simulink model "validacion_LTI"  (R2023b)
settings: Solver=VariableStepAuto  StartTime=0.0  StopTime=10.0  RelTol=1e-3
PostLoadFcn:
  | parametros_sistema_completo
  | run("parametros_sistema_completo.mlx")
values from neighbouring files (symbols this model uses):
  a_cu = 3.9e-3    (= 0.0039)    [parametros_sistema_completo.m]    (also in workspace_params.mat)
  A_sim = sys_design.A    [generar_modelo_LTI.m]
  b_eq = params.b_total    [calcular_matriz_AO.m]    (also in calculo_incertidumbre_y_control.m = b_m + b_l/(r^2); parametros_sistema_completo.m = 2.19444444444e-05; workspace_params.mat = 2.19444444444e-05)
  B_sim = sys_design.B    [generar_modelo_LTI.m]
  C_sim = eye(6)    [generar_modelo_LTI.m]
  C_ts = C_ts * (1 + tol_pct)    [calculo_incertidumbre_y_control.m]    (also in parametros_sistema_completo.m = 0.818; workspace_params.mat = 0.818)
  D_sim = zeros(6,3)    [generar_modelo_LTI.m]
  g = 9.80665    [parametros_sistema_completo.m]    (also in workspace_params.mat)
  J_eq = params.J_total    [calcular_matriz_AO.m]    (also in calculo_incertidumbre_y_control.m = J_m + J_l/r^2; parametros_sistema_completo.m = 1.97847222222e-05; workspace_params.mat = 3.28055555556e-05)
  k_l = m*l_cm + m_l*l_l    [calculo_incertidumbre_y_control.m]    (also in parametros_sistema_completo.m = 0.25; workspace_params.mat = 0.625)
  L_d = L_d    * (1 - tol_pct)    [calculo_incertidumbre_y_control.m]    (also in parametros_sistema_completo.m = 0.0066; workspace_params.mat = 0.0066)
  L_ls = L_ls   * (1 - tol_pct)    [calculo_incertidumbre_y_control.m]    (also in parametros_sistema_completo.m = 0.0008; workspace_params.mat = 0.0008)
  L_q = L_q    * (1 - tol_pct)    [calculo_incertidumbre_y_control.m]    (also in parametros_sistema_completo.m = 0.0058; workspace_params.mat = 0.0058)
  lambda_r = lambda_r * (1 + tol_pct)    [calculo_incertidumbre_y_control.m]    (also in parametros_sistema_completo.m = 0.016; workspace_params.mat = 0.016)
  P_p = 3    [parametros_sistema_completo.m]    (also in workspace_params.mat)
  r = params.r_red    [calcular_matriz_AO.m]    (also in parametros_sistema_completo.m = 120; workspace_params.mat = 120)
  R_sREF = R_sREF * (1 - tol_pct)    [calculo_incertidumbre_y_control.m]    (also in parametros_sistema_completo.m = 1.02; workspace_params.mat = 1.02)
  R_ts_amb = R_ts_amb * (1 - tol_pct)    [calculo_incertidumbre_y_control.m]    (also in parametros_sistema_completo.m = 146.7; workspace_params.mat = 146.7)
  T_amb = 20    [parametros_sistema_completo.m]    (also in workspace_params.mat)
  T_sREF = 20    [parametros_sistema_completo.m]    (also in workspace_params.mat)
  val_th_m_90 = val_th_l_90 * r    [generar_modelo_LTI.m]
settings Model: Creator=Francisco  LastModifiedBy=calde
settings DebuggingCC: UnderspecifiedInitializationDetection=Classic  MergeDetectMultiDrivingBlocksExec=none
settings ModelReferenceCC: PropagateSignalLabelsOutOfModel=off

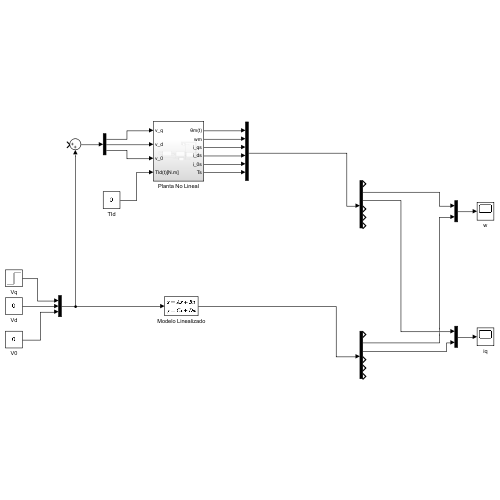
[thumbnail: Simulink's stored preview of the top-level diagram]
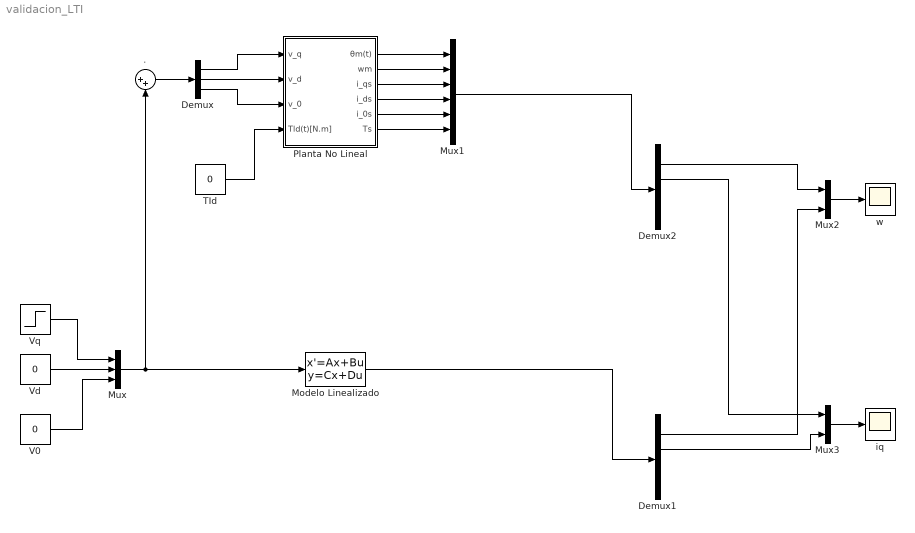
== system validacion_LTI ==
  . : Sum  Inputs=|++
  Demux : Demux  Outputs=3
  Demux1 : Demux  Outputs=6
  Demux2 : Demux  Outputs=6
  Modelo Linealizado : StateSpace  A=A_sim  B=B_sim  C=C_sim  D=D_sim  InitialCondition=0
  Mux : Mux  Inputs=3
  Mux1 : Mux  Inputs=6
  Mux2 : Mux  Inputs=2
  Mux3 : Mux  Inputs=2
  Planta No Lineal : Subsystem
  TId : Constant  Value=0
  V0 : Constant  Value=0
  Vd : Constant  Value=0
  Vq : Step  Time=0.5  SampleTime=0
  iq : Scope
  w : Scope
  wires:
  TId/1 -> Planta No Lineal/4(Tld(t)[N.m])
  Vq/1 -> Mux/1
  Vd/1 -> Mux/2
  V0/1 -> Mux/3
  Mux/1 -> Modelo Linealizado/1, ./2
  ./1 -> Demux/1
  Demux/1 -> Planta No Lineal/1(v_q)
  Demux/2 -> Planta No Lineal/2(v_d)
  Demux/3 -> Planta No Lineal/3(v_0)
  Planta No Lineal/1(θm(t)) -> Mux1/1
  Planta No Lineal/2(wm) -> Mux1/2
  Planta No Lineal/3(i_qs) -> Mux1/3
  Planta No Lineal/4(i_ds) -> Mux1/4
  Planta No Lineal/5(i_0s) -> Mux1/5
  Planta No Lineal/6(Ts) -> Mux1/6
  Mux1/1 -> Demux2/1
  Demux2/2 -> Mux2/1
  Demux2/3 -> Mux3/1
  Demux1/2 -> Mux2/2
  Demux1/3 -> Mux3/2
  Mux2/1 -> w/1
  Mux3/1 -> iq/1
  Modelo Linealizado/1 -> Demux1/1

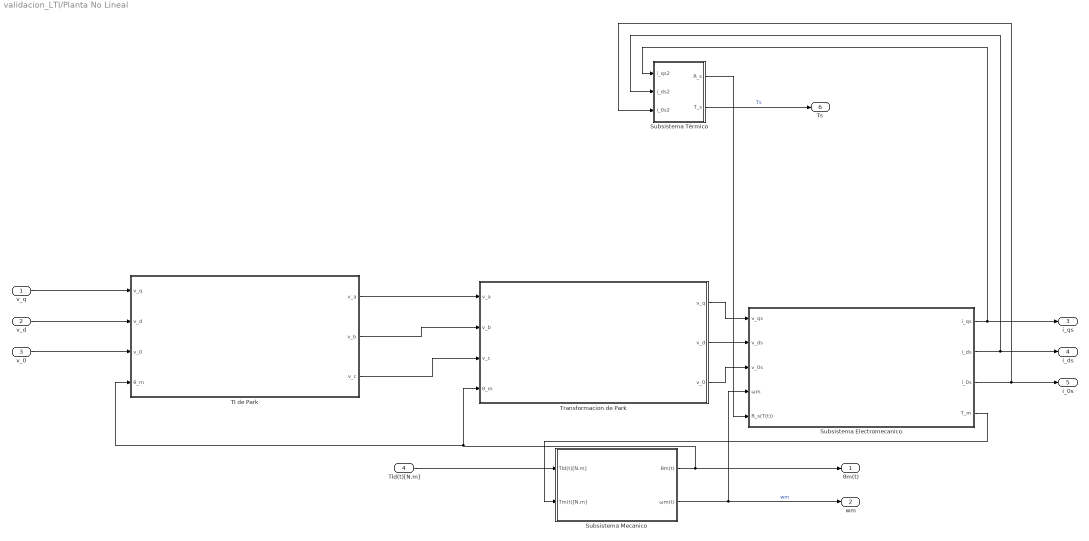
== system validacion_LTI/Planta No Lineal ==
  v_q : Inport
  v_d : Inport  Port=2
  v_0 : Inport  Port=3
  Tld(t)[N.m] : Inport  Port=4
  Subsistema Electromecanico : Subsystem
  Subsistema Mecanico : Subsystem
  Subsistema Térmico : Subsystem
  TI de Park : Subsystem
  Transformacion de Park : Subsystem
  θm(t) : Outport
  wm : Outport  Port=2
  i_qs : Outport  Port=3
  i_ds : Outport  Port=4
  i_0s : Outport  Port=5
  Ts : Outport  Port=6
  wires:
  TI de Park/1(v_a) -> Transformacion de Park/1(v_a)
  TI de Park/3(v_c) -> Transformacion de Park/3(v_c)
  Transformacion de Park/1(v_q) -> Subsistema Electromecanico/1(v_qs)
  TI de Park/2(v_b) -> Transformacion de Park/2(v_b)
  Subsistema Electromecanico/4(T_m) -> Subsistema Mecanico/2(Tm(t)[N.m])
  Subsistema Electromecanico/2(i_ds) -> i_ds/1, Subsistema Térmico/2(i_ds2)
  Subsistema Mecanico/1(θm(t)) -> θm(t)/1, TI de Park/4(θ_m), Transformacion de Park/4(θ_m)
  Subsistema Electromecanico/3(i_0s) -> i_0s/1, Subsistema Térmico/3(i_0s2)
  Subsistema Mecanico/2(ωm(t)) -> wm/1, Subsistema Electromecanico/4(ωm)  "wm"
  Subsistema Térmico/1(R_s) -> Subsistema Electromecanico/5(R_s(T(t)))
  Transformacion de Park/3(v_0) -> Subsistema Electromecanico/3(v_0s)
  Transformacion de Park/2(v_d) -> Subsistema Electromecanico/2(v_ds)
  Subsistema Electromecanico/1(i_qs) -> i_qs/1, Subsistema Térmico/1(i_qs2)
  v_q/1 -> TI de Park/1(v_q)
  v_d/1 -> TI de Park/2(v_d)
  Tld(t)[N.m]/1 -> Subsistema Mecanico/1(Tld(t)[N.m])
  v_0/1 -> TI de Park/3(v_0)
  Subsistema Térmico/2(T_s) -> Ts/1  "Ts"

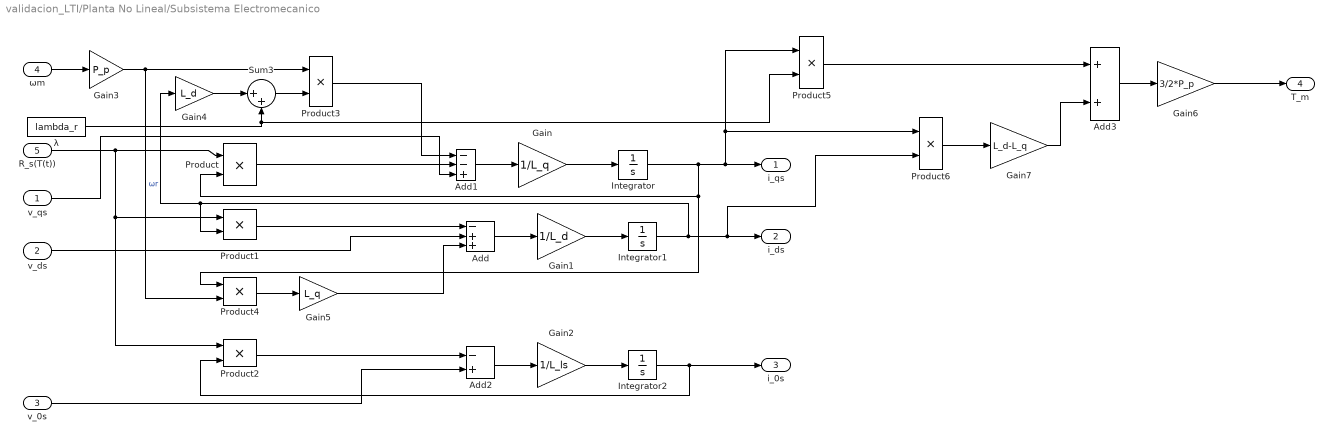
== system validacion_LTI/Planta No Lineal/Subsistema Electromecanico ==
  v_qs : Inport
  v_ds : Inport  Port=2
  v_0s : Inport  Port=3
  ωm : Inport  Port=4
  R_s(T(t)) : Inport  Port=5
  Add : Sum  Inputs=-++
  Add1 : Sum  Inputs=--+
  Add2 : Sum  Inputs=-+
  Add3 : Sum
  Gain : Gain  Gain=1/L_q
  Gain1 : Gain  Gain=1/L_d
  Gain2 : Gain  Gain=1/L_ls
  Gain3 : Gain  Gain=P_p
  Gain4 : Gain  Gain=L_d
  Gain5 : Gain  Gain=L_q
  Gain6 : Gain  Gain=3/2*P_p
  Gain7 : Gain  Gain=L_d-L_q
  Integrator : Integrator
  Integrator1 : Integrator
  Integrator2 : Integrator
  Product{,1..6} (7 alike) : Product
  Sum3 : Sum  Inputs=|++
  λ : Constant  Value=lambda_r
  i_qs : Outport
  i_ds : Outport  Port=2
  i_0s : Outport  Port=3
  T_m : Outport  Port=4
  wires:
  v_0s/1 -> Add2/2
  Gain5/1 -> Add/3
  Gain3/1 -> Product4/2, Product3/1  "ωr"
  Integrator/1 -> Product4/1, Product/2, i_qs/1, Product5/1, Product6/1
  v_qs/1 -> Add1/3
  R_s(T(t))/1 -> Product2/1, Product1/1, Product/1
  Gain4/1 -> Sum3/1
  Product1/1 -> Add/1
  Integrator2/1 -> i_0s/1, Product2/2
  Sum3/1 -> Product3/2
  Integrator1/1 -> Gain4/1, Product1/2, i_ds/1, Product6/2
  Product/1 -> Add1/2
  Product4/1 -> Gain5/1
  ωm/1 -> Gain3/1
  Add3/1 -> Gain6/1
  Gain/1 -> Integrator/1
  Gain6/1 -> T_m/1
  Product2/1 -> Add2/1
  λ/1 -> Sum3/2, Product5/2
  Gain1/1 -> Integrator1/1
  Add/1 -> Gain1/1
  Add1/1 -> Gain/1
  Product6/1 -> Gain7/1
  Product3/1 -> Add1/1
  Gain2/1 -> Integrator2/1
  Gain7/1 -> Add3/2
  v_ds/1 -> Add/2
  Add2/1 -> Gain2/1
  Product5/1 -> Add3/1

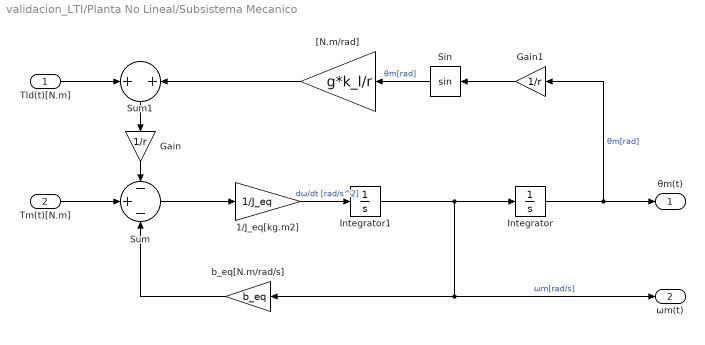
== system validacion_LTI/Planta No Lineal/Subsistema Mecanico ==
  Tld(t)[N.m] : Inport
  Tm(t)[N.m] : Inport  Port=2
  1/J_eq[kg.m2] : Gain  Gain=1/J_eq
  Gain : Gain  Gain=1/r
  Gain1 : Gain  Gain=1/r
  Integrator : Integrator  InitialCondition=val_th_m_90
  Integrator1 : Integrator
  Sin : Trigonometry
  Sum : Sum  Inputs=-+-
  Sum1 : Sum
  "[N.m/rad]" : Gain  Gain=g*k_l/r
  b_eq[N.m/rad/s] : Gain  Gain=b_eq
  θm(t) : Outport
  ωm(t) : Outport  Port=2
  wires:
  Gain1/1 -> Sin/1
  Sin/1 -> "[N.m/rad]"/1  "θm[rad]"
  Integrator1/1 -> Integrator/1, ωm(t)/1, b_eq[N.m/rad/s]/1  "ωm[rad/s]"
  Tld(t)[N.m]/1 -> Sum1/1
  b_eq[N.m/rad/s]/1 -> Sum/3
  1/J_eq[kg.m2]/1 -> Integrator1/1  "dω/dt [rad/s^2]"
  Gain/1 -> Sum/1
  "[N.m/rad]"/1 -> Sum1/2
  Integrator/1 -> θm(t)/1, Gain1/1  "θm[rad]"
  Sum/1 -> 1/J_eq[kg.m2]/1
  Tm(t)[N.m]/1 -> Sum/2
  Sum1/1 -> Gain/1

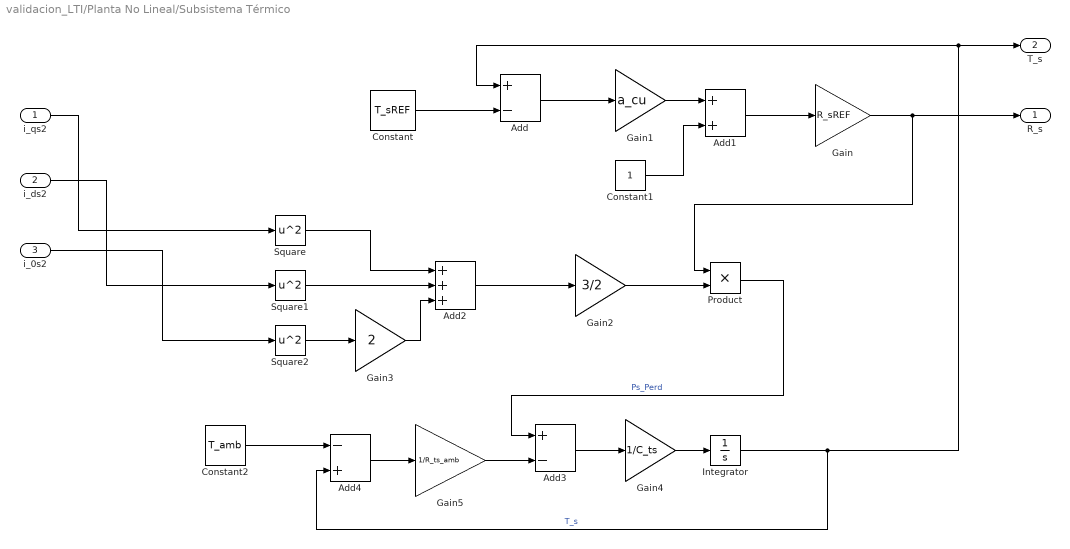
== system validacion_LTI/Planta No Lineal/Subsistema Térmico ==
  i_qs2 : Inport
  i_ds2 : Inport  Port=2
  i_0s2 : Inport  Port=3
  Add : Sum  Inputs=+-
  Add1 : Sum
  Add2 : Sum  Inputs=+++
  Add3 : Sum  Inputs=+-
  Add4 : Sum  Inputs=-+
  Constant : Constant  Value=T_sREF
  Constant1 : Constant
  Constant2 : Constant  Value=T_amb  VectorParams1D=off
  Gain : Gain  Gain=R_sREF
  Gain1 : Gain  Gain=a_cu
  Gain2 : Gain  Gain=3/2
  Gain3 : Gain  Gain=2
  Gain4 : Gain  Gain=1/C_ts
  Gain5 : Gain  Gain=1/R_ts_amb
  Integrator : Integrator  InitialCondition=20
  Product : Product
  Square : Math  Operator=square  OutDataTypeStr=double
  Square1 : Math  Operator=square
  Square2 : Math  Operator=square
  R_s : Outport
  T_s : Outport  Port=2
  wires:
  Constant1/1 -> Add1/2
  Constant/1 -> Add/2
  i_qs2/1 -> Square/1
  Gain/1 -> R_s/1, Product/1
  Square/1 -> Add2/1
  Add2/1 -> Gain2/1
  Constant2/1 -> Add4/1
  i_ds2/1 -> Square1/1
  Gain5/1 -> Add3/2
  Integrator/1 -> Add4/2, T_s/1, Add/1  "T_s"
  Add1/1 -> Gain/1
  i_0s2/1 -> Square2/1
  Square1/1 -> Add2/2
  Product/1 -> Add3/1  "Ps_Perd"
  Gain2/1 -> Product/2
  Add/1 -> Gain1/1
  Square2/1 -> Gain3/1
  Gain1/1 -> Add1/1
  Add3/1 -> Gain4/1
  Add4/1 -> Gain5/1
  Gain3/1 -> Add2/3
  Gain4/1 -> Integrator/1

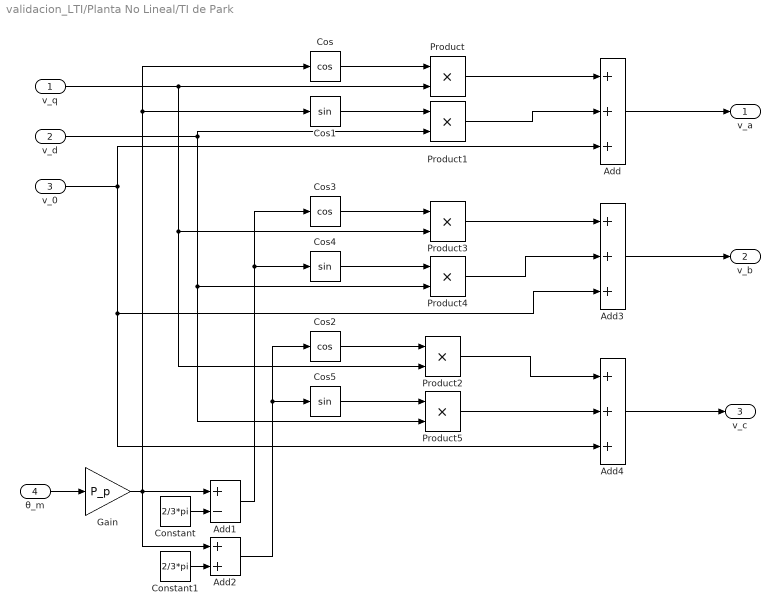
== system validacion_LTI/Planta No Lineal/TI de Park ==
  v_q : Inport
  v_d : Inport  Port=2
  v_0 : Inport  Port=3
  θ_m : Inport  Port=4
  Add : Sum  Inputs=+++
  Add1 : Sum  Inputs=+-
  Add2 : Sum
  Add3 : Sum  Inputs=+++
  Add4 : Sum  Inputs=+++
  Constant : Constant  Value=2/3*pi
  Constant1 : Constant  Value=2/3*pi
  Cos : Trigonometry  Operator=cos
  Cos1 : Trigonometry
  Cos2 : Trigonometry  Operator=cos
  Cos3 : Trigonometry  Operator=cos
  Cos4 : Trigonometry
  Cos5 : Trigonometry
  Gain : Gain  Gain=P_p
  Product{,1..5} (6 alike) : Product
  v_a : Outport
  v_b : Outport  Port=2
  v_c : Outport  Port=3
  wires:
  Product4/1 -> Add3/2
  Cos1/1 -> Product1/1
  Cos/1 -> Product/1
  Product1/1 -> Add/2
  Add3/1 -> v_b/1
  Cos3/1 -> Product3/1
  Product3/1 -> Add3/1
  v_d/1 -> Product1/2, Product5/2, Product4/2
  Constant1/1 -> Add2/2
  Constant/1 -> Add1/2
  v_0/1 -> Add3/3, Add4/3, Add/3
  Add1/1 -> Cos3/1, Cos4/1
  Product/1 -> Add/1
  v_q/1 -> Product/2, Product2/2, Product3/2
  Cos4/1 -> Product4/1
  Gain/1 -> Add2/1, Add1/1, Cos/1, Cos1/1
  θ_m/1 -> Gain/1
  Add/1 -> v_a/1
  Add4/1 -> v_c/1
  Cos2/1 -> Product2/1
  Cos5/1 -> Product5/1
  Add2/1 -> Cos5/1, Cos2/1
  Product2/1 -> Add4/1
  Product5/1 -> Add4/2

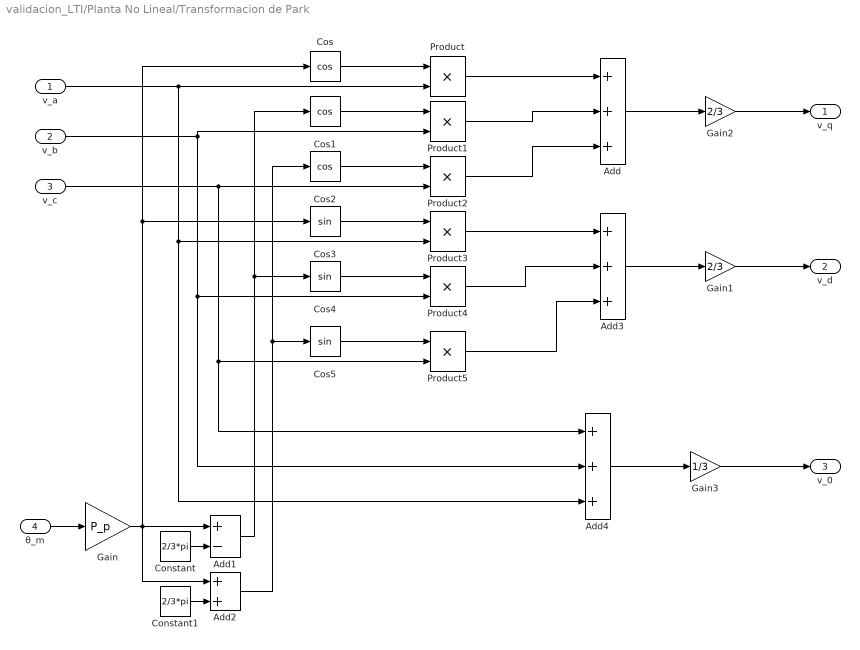
== system validacion_LTI/Planta No Lineal/Transformacion de Park ==
  v_a : Inport
  v_b : Inport  Port=2
  v_c : Inport  Port=3
  θ_m : Inport  Port=4
  Add : Sum  Inputs=+++
  Add1 : Sum  Inputs=+-
  Add2 : Sum
  Add3 : Sum  Inputs=+++
  Add4 : Sum  Inputs=+++
  Constant : Constant  Value=2/3*pi
  Constant1 : Constant  Value=2/3*pi
  Cos : Trigonometry  Operator=cos
  Cos1 : Trigonometry  Operator=cos
  Cos2 : Trigonometry  Operator=cos
  Cos3 : Trigonometry
  Cos4 : Trigonometry
  Cos5 : Trigonometry
  Gain : Gain  Gain=P_p
  Gain1 : Gain  Gain=2/3
  Gain2 : Gain  Gain=2/3
  Gain3 : Gain  Gain=1/3
  Product{,1..5} (6 alike) : Product
  v_q : Outport
  v_d : Outport  Port=2
  v_0 : Outport  Port=3
  wires:
  θ_m/1 -> Gain/1
  Cos5/1 -> Product5/1
  Gain2/1 -> v_q/1
  Product5/1 -> Add3/3
  Add/1 -> Gain2/1
  Gain/1 -> Cos3/1, Cos/1, Add1/1, Add2/1
  Cos4/1 -> Product4/1
  Cos2/1 -> Product2/1
  v_a/1 -> Add4/3, Product3/2, Product/2
  Product/1 -> Add/1
  Add1/1 -> Cos1/1, Cos4/1
  v_c/1 -> Product2/2, Product5/2, Add4/1
  Constant/1 -> Add1/2
  Constant1/1 -> Add2/2
  v_b/1 -> Product1/2, Product4/2, Add4/2
  Add2/1 -> Cos2/1, Cos5/1
  Add4/1 -> Gain3/1
  Product3/1 -> Add3/1
  Product2/1 -> Add/3
  Gain3/1 -> v_0/1
  Cos3/1 -> Product3/1
  Add3/1 -> Gain1/1
  Gain1/1 -> v_d/1
  Product1/1 -> Add/2
  Cos/1 -> Product/1
  Cos1/1 -> Product1/1
  Product4/1 -> Add3/2
